simulink model "ball_nozerocross"  (Simulink 4.00)
settings: Solver=ode45  StartTime=0.0  StopTime=8  RelTol=1e-2
settings Model: LastModifiedBy=hespanha  ZeroCross=off  BlockReductionOpt=off

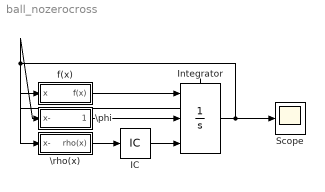
== system ball_nozerocross ==
  IC : InitialCondition  Value=[10;5]
  Integrator : Integrator  ExternalReset=rising  InitialConditionSource=external  InitialCondition=0  LimitOutput=off  UpperSaturationLimit=inf  LowerSaturationLimit=-inf  ShowSaturationPort=off  ShowStatePort=on  AbsoluteTolerance=auto
  Scope : Scope
      settings: TimeRange=8  YMin=-15  YMax=15  SaveToWorkspace=off  SaveName=ScopeData  LimitDataPoints=on  MaxDataPoints=5000
  \phi : Subsystem  Description=f(x)
      settings: RTWFcnNameOpts=Auto  RTWFileNameOpts=Auto
  \rho(x) : Subsystem  Description=f(x)
      settings: RTWFcnNameOpts=Auto  RTWFileNameOpts=Auto
  f(x) : Subsystem  Description=f(x)
      settings: RTWFcnNameOpts=Auto  RTWFileNameOpts=Auto
  wires:
  IC/1 -> Integrator/3
  f(x)/1(f(x)) -> Integrator/1
  \phi/1(x\in\phi) -> Integrator/2
  Integrator/State -> \rho(x)/1(x-), \phi/1(x-)
  \rho(x)/1(rho(x)) -> IC/1
  Integrator/1 -> f(x)/1(x), Scope/1

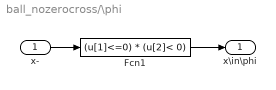
== system ball_nozerocross/\phi ==
  x- : Inport  Port=1
  Fcn1 : Fcn  Expr=(u[1]<=0) * (u[2]< 0)
  x\in\phi : Outport  Port=1
  wires:
  x-/1 -> Fcn1/1
  Fcn1/1 -> x\in\phi/1

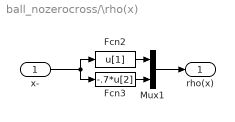
== system ball_nozerocross/\rho(x) ==
  x- : Inport  Port=1
  Fcn2 : Fcn  Expr=u[1]
  Fcn3 : Fcn  Expr=-.7*u[2]
  Mux1 : Mux  Inputs=2
  rho(x) : Outport  Port=1
  wires:
  Fcn3/1 -> Mux1/2
  Fcn2/1 -> Mux1/1
  Mux1/1 -> rho(x)/1
  x-/1 -> Fcn2/1, Fcn3/1

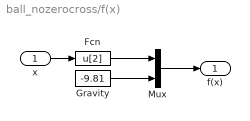
== system ball_nozerocross/f(x) ==
  x : Inport  Port=1
  Fcn : Fcn  Expr=u[2]
  Gravity : Constant  Value=-9.81
  Mux : Mux  Inputs=2
  f(x) : Outport  Port=1
  wires:
  Mux/1 -> f(x)/1
  Gravity/1 -> Mux/2
  Fcn/1 -> Mux/1
  x/1 -> Fcn/1
